simulink subsystem "DCFaulhaber"  (R2023b)
settings: Solver=VariableStepAuto  StartTime=0.0  StopTime=10.0  RelTol=1e-3
libraries: ee_lib x1, fl_lib x1
settings Model: DataDictionary=neck_mk3.sldd  EnableAccessToBaseWorkspace=off  Creator=upattacini  LastModifiedBy=upattacini

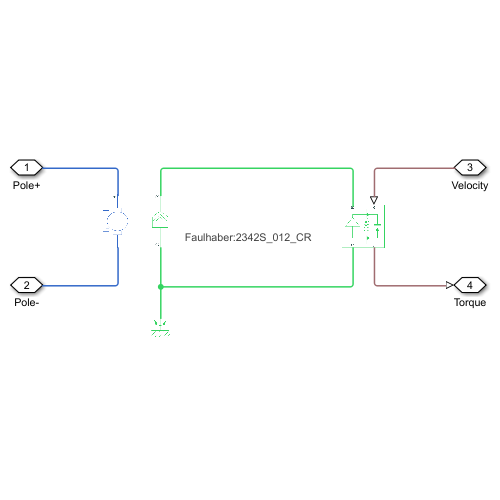
[thumbnail: Simulink's stored preview of the top-level diagram]
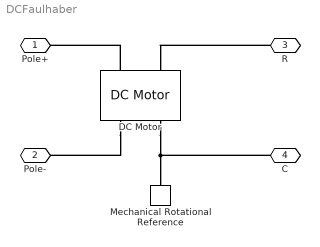
== system DCFaulhaber ==
  DC Motor : ee_lib/Electromechanical/Brushed Motors/DC Motor  Tag={'toolbox/physmod/elec/library/m/ee_lib_parts';'Electromechanical/Brushed_Motors/DC_Motor/Faulhaber/x2342S_012_CR.xml'}  field_option=ee.enum.field_option.pm  Rf=100 % Parameter not set Ohm  Lf=1 % Parameter not set H  Laf=0.15 % Parameter not set H  If0=0 % Parameter not set A  parameterization=ee.enum.dcparam_option.circuit_param  Ra=1.9 Ohm  La=0.065 mH  emf_or_torque=ee.enum.emf_or_torque.ki  Kv=1.40324 % Parameter estimated mV/rpm  Ki=13.4 mN*m/A  T_stall=0.24e-3 % Parameter not set N*m  w_max=19100 % Parameter not set rpm  w_rated=15000 % Parameter not set rpm  P_rated=0.08 % Parameter not set W  V_rated=1.5 % Parameter not set V  lam_param=ee.enum.lam_param.current  i_noload=0.075 A  V_i_noload=Vcc V  J=5.7 g*cm^2  lam=0 % % Parameter not set mN*m/(rad/s)  speed0=0 % Parameter not set rpm  enable_fault_armature=simscape.enum.onoff.off  rev_faulted=1 / 3 % Parameter not set  G_faulted_armature=1e-5 % Parameter not set S  fault_trigger_armature=ee.enum.faults.faultTrigger.temporal  t_fault_armature=1 % Parameter not set s  max_permissible_current_armature=inf % Parameter not set A  t_fail_on_current_armature=1 % Parameter not set s  enable_fault_field=simscape.enum.onoff.off  G_faulted_field=1e-5 % Parameter not set S  fault_trigger_field=ee.enum.faults.faultTrigger.temporal  t_fault_field=1 % Parameter not set s  max_permissible_current_field=inf % Parameter not set A  t_fail_on_current_field=1 % Parameter not set s  fault_action=simscape.enum.assert.action.none  alpha=3.93e-3 1/K  Tmeas=25 degC  thermal_mass=100 J/K  initial_temperature=25 degC
      settings: AttributesFormatString=Faulhaber:2342S_012_CR
  Mechanical Rotational Reference : fl_lib/Mechanical/Rotational Elements/Mechanical Rotational Reference
  Pole+ : PMIOPort  Side=Left
  Pole- : PMIOPort  Port=2  Side=Left
  R : PMIOPort  Port=3  Side=Right
  C : PMIOPort  Port=4  Side=Right
  connections:
  C/RConn1 -- DC Motor/RConn2 -- Mechanical Rotational Reference/LConn1
  DC Motor/LConn1 -- Pole+/RConn1
  DC Motor/RConn1 -- Pole-/RConn1
  R/RConn1 -- DC Motor/LConn2
